simulink model "motor_voltageControl_Simulation"  (R2018a)
settings: Solver=VariableStepAuto  StartTime=0.0  StopTime=2  RelTol=1e-3
values from neighbouring files (symbols this model uses):
  c_r = 2.5e-6    (= 2.5e-06)    [lab03_part01.m]    (also in lab06_simulationWithMeasurements.m = 1.15e-06)
  J = 5.5e-6    (= 5.5e-06)    [lab03_part01.m]    (also in lab04_part01.m = 8e-06; lab05_part01_baga.m = 8e-06; lab06_simulationWithMeasurements.m = 5.29e-06)
  k_e = 23.7e-3    (= 0.0237)    [lab03_part01.m]    (also in lab06_simulationWithMeasurements.m = 0.02375)
  k_m = 22.46e-3    (= 0.02246)    [lab03_part01.m]    (also in lab06_simulationWithMeasurements.m)
  L = tan(phi).*Rges./(frequencies.*2*pi)    [lab02_part01.m]    (also in lab03_part01.m = 0.0005752; lab04_part01.m = 0.00035329; lab05_part01_baga.m = 0.00035329; lab06_simulationWithMeasurements.m = 0.000618)
  R_A = 3.22    [lab03_part01.m]    (also in lab05_part01_baga.m = 3.71; lab06_simulationWithMeasurements.m)
  R_S = 1    [lab03_part01.m]    (also in lab05_part01_baga.m; lab06_simulationWithMeasurements.m)
  U0 = 10    [lab03_part01.m]
settings Model: Creator=oleksandra  LastModifiedBy=oleksandra

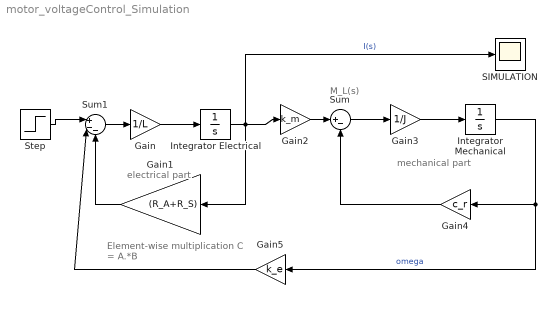
== system motor_voltageControl_Simulation ==
  note: M_L(s)
  note: Element-wise multiplication C = A.*B
  note: electrical part
  note: mechanical part
  Gain : Gain  Gain=1/L  SaturateOnIntegerOverflow=on  OutDataTypeStr=Inherit: Same as input  ParamDataTypeStr=Inherit: Same as input
  Gain1 : Gain  Gain=(R_A+R_S)  SaturateOnIntegerOverflow=on  OutDataTypeStr=Inherit: Same as input  ParamDataTypeStr=Inherit: Same as input
  Gain2 : Gain  Gain=k_m  SaturateOnIntegerOverflow=on  OutDataTypeStr=Inherit: Same as input  ParamDataTypeStr=Inherit: Same as input
  Gain3 : Gain  Gain=1/J  SaturateOnIntegerOverflow=on  OutDataTypeStr=Inherit: Same as input  ParamDataTypeStr=Inherit: Same as input
  Gain4 : Gain  Gain=c_r  SaturateOnIntegerOverflow=on  OutDataTypeStr=Inherit: Same as input  ParamDataTypeStr=Inherit: Same as input
  Gain5 : Gain  Gain=k_e  SaturateOnIntegerOverflow=on  OutDataTypeStr=Inherit: Same as input  ParamDataTypeStr=Inherit: Same as input
  Integrator Electrical : Integrator
  Integrator Mechanical : Integrator
  SIMULATION : Scope
  Step : Step  Time=0.1  After=U0  SampleTime=0
  Sum : Sum  Inputs=|+-  SaturateOnIntegerOverflow=on  InputSameDT=on  OutDataTypeStr=Inherit: Same as first input
  Sum1 : Sum  Inputs=|+--  SaturateOnIntegerOverflow=on  InputSameDT=on  OutDataTypeStr=Inherit: Same as first input
  wires:
  Integrator Electrical/1 -> SIMULATION/1, Gain2/1, Gain1/1  "I(s)"
  Gain2/1 -> Sum/1
  Gain5/1 -> Sum1/2
  Gain1/1 -> Sum1/3
  Step/1 -> Sum1/1
  Gain4/1 -> Sum/2
  Integrator Mechanical/1 -> Gain4/1, Gain5/1  "omega"
  Sum1/1 -> Gain/1
  Gain/1 -> Integrator Electrical/1
  Gain3/1 -> Integrator Mechanical/1
  Sum/1 -> Gain3/1
